simulink model "Model_SimpleThermal_14b"  (R2014b)
settings: Solver=ode45  StartTime=0.0  StopTime=10.0  RelTol=1e-3
undefined symbols (not defined in the file or in its folder): in, param
settings Model: Creator=Arek  LastModifiedBy=Arek
settings SolverCC: ZeroCrossAlgorithm=Adaptive

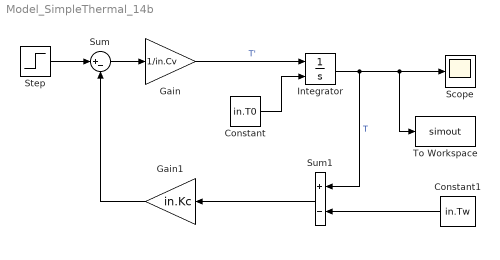
== system Model_SimpleThermal_14b ==
  Constant : Constant  Value=in.T0
  Constant1 : Constant  Value=in.Tw
  Gain : Gain  Gain=1/in.Cv
  Gain1 : Gain  Gain=in.Kc
  Integrator : Integrator  InitialConditionSource=external  InitialCondition=in.T0
  Scope : Scope
  Step : Step  Time=param.tstart  After=in.qN  SampleTime=0
  Sum : Sum  Inputs=|+-
  Sum1 : Sum  Inputs=+-
  To Workspace : ToWorkspace  VariableName=simout  SaveFormat=Timeseries  SampleTime=-1
  wires:
  Constant/1 -> Integrator/2
  Gain/1 -> Integrator/1  "T'"
  Integrator/1 -> To Workspace/1, Scope/1, Sum1/1  "T"
  Sum/1 -> Gain/1
  Gain1/1 -> Sum/2
  Sum1/1 -> Gain1/1
  Constant1/1 -> Sum1/2
  Step/1 -> Sum/1
